simulink model "example_GPF"  (R2016a)
settings: Solver=VariableStepAuto  StartTime=0.0  StopTime=20  RelTol=1e-3
undefined symbols (not defined in the file): KFparam, Ts
settings Model: Creator=mgreiff  LastModifiedBy=mgreiff
settings DataIOCC: LimitDataPoints=on
settings DebuggingCC: AllowSymbolicDim=off
settings ModelReferenceCC: PropagateSignalLabelsOutOfModel=off
settings GRTTargetCC: GeneratePreprocessorConditionals=Use local settings

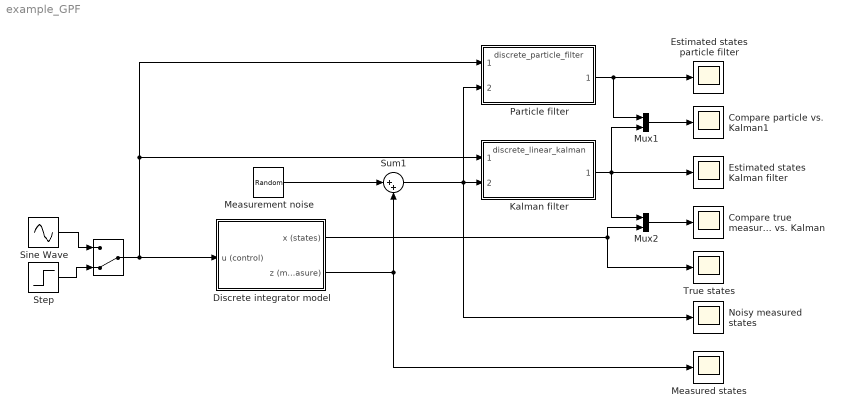
== system example_GPF ==
  " " : ManualSwitch  CurrentSetting=0
  Compare particle vs. Kalman1 : Scope
  Compare true measurements vs. Kalman : Scope
  Discrete integrator model : Subsystem
  Estimated states Kalman filter : Scope
  Estimated states particle filter : Scope
  Kalman filter : ModelReference  ModelNameDialog=discrete_linear_kalman.slx  SimulationMode=Normal  ModelReferenceVersion=1.93
  Measured states : Scope
  Measurement noise : RandomNumber  Variance=KFparam.std_R^2  SampleTime=Ts
  Mux1 : Mux  Inputs=2
  Mux2 : Mux  Inputs=2
  Noisy measured states : Scope
  Particle filter : ModelReference  ModelNameDialog=discrete_particle_filter.slx  SimulationMode=Normal  ModelReferenceVersion=1.15
  Sine Wave : Sin  SampleTime=0
  Step : Step  SampleTime=0
  Sum1 : Sum  Inputs=|++
  True states : Scope
  wires:
  " "/1 -> Kalman filter/1, Particle filter/1, Discrete integrator model/1(u (control))
  Kalman filter/1 -> Mux2/1, Estimated states Kalman filter/1, Mux1/2
  Sum1/1 -> Noisy measured states/1, Particle filter/2, Kalman filter/2
  Measurement noise/1 -> Sum1/1
  Sine Wave/1 -> " "/1
  Step/1 -> " "/2
  Particle filter/1 -> Mux1/1, Estimated states particle filter/1
  Mux1/1 -> Compare particle vs. Kalman1/1
  Mux2/1 -> Compare true measurements vs. Kalman/1
  Discrete integrator model/1(x (states)) -> True states/1, Mux2/2
  Discrete integrator model/2(z (measure)) -> Measured states/1, Sum1/2

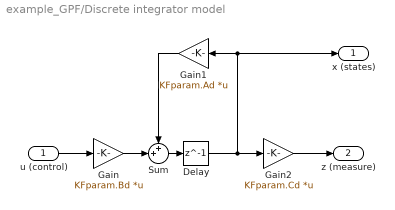
== system example_GPF/Discrete integrator model ==
  u (control) : Inport
  Delay : Delay  DelayLength=1  InitialCondition=0  SampleTime=Ts
  Gain : Gain  Gain=KFparam.Bd  Multiplication=Matrix(K*u)
  Gain1 : Gain  Gain=KFparam.Ad  Multiplication=Matrix(K*u)
  Gain2 : Gain  Gain=KFparam.Cd  Multiplication=Matrix(K*u)
  Sum : Sum  Inputs=++|
  x (states) : Outport
  z (measure) : Outport  Port=2
  wires:
  u (control)/1 -> Gain/1
  Delay/1 -> Gain2/1, x (states)/1, Gain1/1
  Sum/1 -> Delay/1
  Gain1/1 -> Sum/1
  Gain2/1 -> z (measure)/1
  Gain/1 -> Sum/2
